simulink library "Librairie"  (R2015b)
settings: Solver=ode45  StartTime=0.0  StopTime=10.0  RelTol=1e-3
undefined symbols (not defined in the file): fdesignblkfcn, gcbh
libraries: dspsrcs4 x2, dspvision x2, dsparch4 x1, dspsnks4 x1, dspspect3 x1, dspsigops x1
settings Model: Creator=sylar  LastModifiedBy=argentieri
settings DataIOCC: SaveFormat=Array
settings DebuggingCC: AllowSymbolicDim=on
settings HardwareCC: ProdBitPerPointer=32  ProdLargestAtomicFloat=None  ProdIntDivRoundTo=Undefined  ProdEndianess=Unspecified  ProdWordSize=32  ProdHWDeviceType=32-bit Generic
settings GRTTargetCC: GeneratePreprocessorConditionals=Disable all
settings ConfigComp: CovModelRefEnable=Off

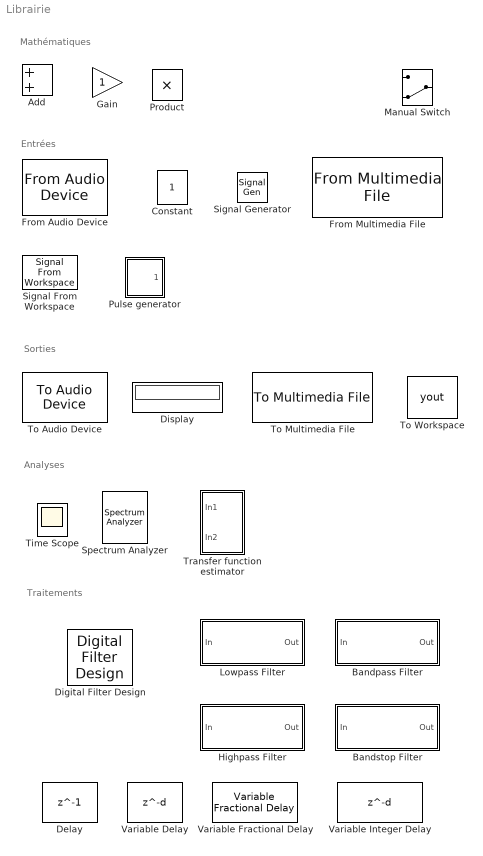
== system Librairie ==
  note: Traitements
  note: Analyses
  note: Sorties
  note: Entrées
  note: Mathématiques
  Add : Sum
  Bandpass Filter : Subsystem  DialogController=fdesignblkfcn  InitFcn=fdesignblkfcn(gcbh, {'InitFcn'});  mask(Bandpass Filter){}
      mask help: Design a bandpass filter
      settings: CopyFcn=fdesignblkfcn(gcbh, {'CopyFcn'});
      mask Help: helpview(mapfilelocation('dsp'), 'dspbandpassfilter');
      mask Display: disp('Bandpass');
  Bandstop Filter : Subsystem  DialogController=fdesignblkfcn  InitFcn=fdesignblkfcn(gcbh, {'InitFcn'});  mask(Bandstop Filter){}
      mask help: Design a bandstop filter
      settings: CopyFcn=fdesignblkfcn(gcbh, {'CopyFcn'});
      mask Help: helpview(mapfilelocation('dsp'), 'dspbandstopfilter');
      mask Display: disp('Bandstop');
  Constant : Constant  VectorParams1D=off
  Delay : Delay  DelayLength=1  DelayLengthUpperLimit=5000  InputProcessing=Columns as channels (frame based)
  Digital Filter Design : dsparch4/Digital Filter Design  mwdsp_browser_bugfix_var=off
  Display : Display
  From Audio Device : dspsrcs4/From Audio Device  deviceName=Default  numChannels=2  sampleRate=A_COMPLETER  deviceDatatype=Determine from output data type  autoBufferSize=on  bufferSize=4096  queueDuration=1.0  frameSize=1024  outputDatatype=double  defaultInputChannelMapping=on  inputChannelMapping=1:2  outputNumOverrunSamples=off  OutputFrames=on
  From Multimedia File : dspvision/From Multimedia File  inputFilename=speech_dft.mp3  loop=on  numPlays=inf  outputStreams=Audio only  videoDataType=single  audioDataType=double  inheritSampleTime=on  userDefinedSampleTime=1/30  noAudioOutput=off  isIntensityVideo=off  fourcc=RGB  colorVideoFormat=Separate color signals  outputEOF=off  dataOrg=Column-major  audioFrameSize=1024  computeAudioFrameSize=off  outSamplingMode=Sample based
  Gain : Gain
  Highpass Filter : Subsystem  DialogController=fdesignblkfcn  InitFcn=fdesignblkfcn(gcbh, {'InitFcn'});  mask(Highpass Filter){}
      mask help: Design a highpass filter
      settings: CopyFcn=fdesignblkfcn(gcbh, {'CopyFcn'});
      mask Help: helpview(mapfilelocation('dsp'), 'dsphighpassfilter');
      mask Display: disp('Highpass')
  Lowpass Filter : Subsystem  DialogController=fdesignblkfcn  InitFcn=fdesignblkfcn(gcbh, {'InitFcn'});  mask(Lowpass Filter){}
      mask help: Design a lowpass filter
      settings: CopyFcn=fdesignblkfcn(gcbh, {'CopyFcn'});
      mask Help: helpview(mapfilelocation('dsp'), 'dsplowpassfilter');
      mask Display: disp('Lowpass')
  Manual Switch : ManualSwitch  CurrentSetting=0
  Product : Product
  Pulse generator : Subsystem  mask{fee=11025, NN=1024}
      mask prompts: fee "fe"; NN "buffer"
      mask DialogControl DescTextVar Prompt: Générateur d'impulsions
      mask Display: port_label('output',1,'out')
  Signal Generator : SignalGenerator  Units=rad/sec
  Signal From Workspace : dspsrcs4/Signal From Workspace  X=1:10  Ts=1  nsamps=1  OutputAfterFinalValue=Setting to zero  ignoreOrWarnInputAndFrameLengths=off  OutputFrames=on
  Spectrum Analyzer : SpectrumAnalyzer
  Time Scope : Scope  NumInputPorts=2
  To Audio Device : dspsnks4/To Audio Device  deviceName=Default  inheritSampleRate=on  sampleRate=44100  deviceDatatype=Determine from input data type  autoBufferSize=on  bufferSize=4096  queueDuration=1.0  defaultOutputChannelMapping=on  outputChannelMapping=1:2  outputNumUnderrunSamples=off
  To Multimedia File : dspvision/To Multimedia File  outputFilename=output.wav  streamSelection=Audio only  videoCompressor=None (uncompressed)  audioCompressor=None (uncompressed)  imagePorts=Separate color signals  fileType=WAV  audioDatatype=16-bit integer  fourcc=RGB  videoQuality=75  mj2000CompFactor=10
  To Workspace : ToWorkspace  VariableName=yout  SampleTime=-1
      settings: Save2DSignal=2-D array (concatenate along first dimension)
  Transfer function estimator : Subsystem  InitFcn=|  mask{fee=11025, NN=1024}
      | name=gcb;
      | p = Simulink.Mask.get(name);
      | fe_tf = str2double(p.getParameter('fee').Value);
      | N_tf = str2double(p.getParameter('NN').Value);
      mask prompts: fee "fe"; NN "N"
      mask init:
      | fs = fee;
      mask Display:
      | port_label('input',1,'in')
      | port_label('input',2,'out')
  Variable Fractional Delay : dspsigops/Variable Fractional Delay  mode=OBSOLETE  modeActive=Linear  dmax=100  InputProcessing=Columns as channels (frame based)  L=4  FarrowL=4  R=10  alpha=1  ic=0  fallbackFIR=Clip to the minimum value necessary for centered kernel  fallbackFarrow=Clip to the minimum value necessary for centered kernel  noDFT=off  roundingMode=Zero  overflowMode=off
  Variable Delay : Delay  DelayLengthSource=Input port  DelayLength=1  DelayLengthUpperLimit=5000  PreventDirectFeedthrough=on  RemoveProtectionDelayLength=on  InputProcessing=Columns as channels (frame based)
      settings: InputPortMap=u0,p1
  Variable Integer Delay : Delay  DelayLengthSource=Input port  InputProcessing=Columns as channels (frame based)
      settings: InputPortMap=u0,p1

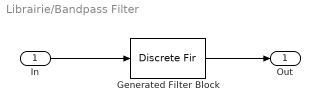
== system Librairie/Bandpass Filter ==
  In : Inport
  Generated Filter Block : DiscreteFir  Tag=BlockMethodSubSystem  Coefficients=[0.00145487204688885528 -0.0257757164809061523 -0.0154961019891340819 0.0344439493870172947 0.0115097335885992382 0.020748633693885337 0.0863287912807311486 -0.08086143736002184 -0.265551029631479307 0.050017971996636254 0.36058953309117231 0.050017971996636254 -0.265551029631479307 -0.08086143736002184 0.0863287912807311486 0.020748633693885337 0.0115097335885992382 0.0344439493870172947 -0.0154961019891340819 -0.0257757164809061523 0.00145487204688885528]  InputProcessing=Columns as channels (frame based)
  Out : Outport
  wires:
  In/1 -> Generated Filter Block/1
  Generated Filter Block/1 -> Out/1

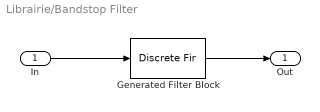
== system Librairie/Bandstop Filter ==
  In : Inport
  Generated Filter Block : DiscreteFir  Tag=BlockMethodSubSystem  Coefficients=[0.068428203108407068 -0.112824153131554777 -0.095934196931819149 -0.0678357126098109581 -0.0120668492639047983 0.0507019014458022152 0.0839729096350368548 0.0648109769310018374 0.00226627607110810184 -0.0646907037212710589 0.906667314762344412 -0.0646907037212710589 0.00226627607110810184 0.0648109769310018374 0.0839729096350368548 0.0507019014458022152 -0.0120668492639047983 -0.0678357126098109581 -0.095934196931819149 -0.112824153131554777 0.068428203108407068]  InputProcessing=Columns as channels (frame based)
  Out : Outport
  wires:
  Generated Filter Block/1 -> Out/1
  In/1 -> Generated Filter Block/1

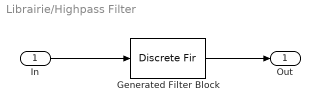
== system Librairie/Highpass Filter ==
  In : Inport
  Generated Filter Block : DiscreteFir  Tag=BlockMethodSubSystem  Coefficients=[0.0209800180162859756 -0.0206132779322321172 -0.023413586493171764 -0.00982538427506522705 0.022656337288466652 0.0514623626939051115 0.0407037090513912014 -0.0308156127751440558 -0.146545018650288961 -0.254897103724912921 0.700803760913058404 -0.254897103724912921 -0.146545018650288961 -0.0308156127751440558 0.0407037090513912014 0.0514623626939051115 0.022656337288466652 -0.00982538427506522705 -0.023413586493171764 -0.0206132779322321172 0.0209800180162859756]  InputProcessing=Columns as channels (frame based)
  Out : Outport
  wires:
  Generated Filter Block/1 -> Out/1
  In/1 -> Generated Filter Block/1

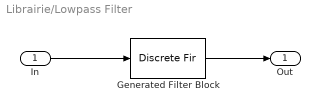
== system Librairie/Lowpass Filter ==
  In : Inport
  Generated Filter Block : DiscreteFir  Tag=BlockMethodSubSystem  Coefficients=[2.50606596102242362e-05 -0.000137613798736198572 0.000163370767243491345 0.000214028644429250798 -0.000211749055172579648 -0.000651442325393265624 -7.16938181093962606e-05 0.00133502830784752052 0.00140186203480473313 -0.0012801418811304022 -0.00393791878592938006 -0.00160266048757988044 0.00540316118214430752 0.00831949252759633245 -0.000601061894001873355 -0.0144745350808635556 -0.0140886818018923759 0.00873958063312104023 0.0320448163395401081 0.0200657121962688478 -0.0312907115777847147 -0.0698595105093784557 -0.0246182818742873705 0.119412911224633433 0.285872391089864453 0.359657172755037335 0.285872391089864453 0.119412911224633433 -0.0246182818742873705 -0.0698595105093784557 -0.0312907115777847147 0.0200657121962688478 0.0320448163395401081 0.00873958063312104023 -0.0140886818018923759 -0.0144745350808635556 -0.000601061894001873355 0.00831949252759633245 0.00540316118214430752 -0.00160266048757988044 -0.00393791878592938006 -0.0012801418811304022 0.00140186203480473313 0.00133502830784752052 -7.16938181093962606e-05 -0.000651442325393265624 -0.000211749055172579648 0.000214028644429250798 0.000163370767243491345 -0.000137613798736198572 2.50606596102242362e-05]  InputProcessing=Columns as channels (frame based)
  Out : Outport
  wires:
  In/1 -> Generated Filter Block/1
  Generated Filter Block/1 -> Out/1

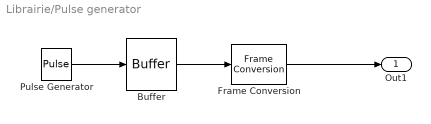
== system Librairie/Pulse generator ==
  Buffer : Buffer  N=NN  TreatMby1Signals=One channel  OutputFrames=off
  Frame Conversion : FrameConversion  InheritSamplingMode=off
  Pulse Generator : DiscretePulseGenerator  Period=NN  SampleTime=1/fee
  Out1 : Outport
  wires:
  Buffer/1 -> Frame Conversion/1
  Pulse Generator/1 -> Buffer/1
  Frame Conversion/1 -> Out1/1

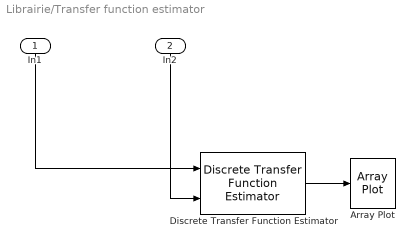
== system Librairie/Transfer function estimator ==
  In1 : Inport
  In2 : Inport  Port=2
  Array Plot : ArrayPlot
  Discrete Transfer Function Estimator : dspspect3/Discrete Transfer Function Estimator  WindowMode=Specify on dialog  WindowLength=NN  Overlap=50  SpectralAverages=100  FFTLengthSource=Auto  FFTLength=128  Window=Hann  SidelobeAttenuation=60  FrequencyRange=One-sided  OutputCoherence=off  SimulateUsing=Code generation
  wires:
  In2/1 -> Discrete Transfer Function Estimator/2
  In1/1 -> Discrete Transfer Function Estimator/1
  Discrete Transfer Function Estimator/1 -> Array Plot/1
